simulink model "behavior_IMM_Pred"  (R2019b)
settings: Solver=FixedStepAuto  StartTime=0.0  StopTime=25  FixedStep=Ts_bp  RelTol=1e-3
undefined symbols (not defined in the file or in its folder): P_init, sigbuilder_block, Ts_bp, vx, vy, x, y
libraries: simulink x2
settings Model: Creator=jasprit  LastModifiedBy=jasprit

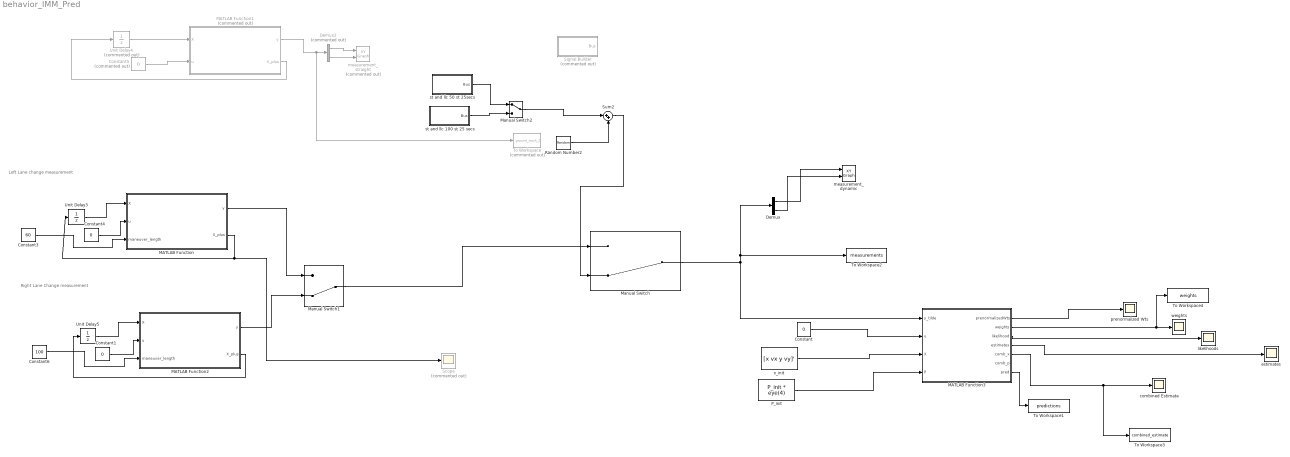
== system behavior_IMM_Pred ==
  note: Left Lane change measurement
  note: Right Lane Change measurement
  Constant : Constant  Value=0
  Constant1 : Constant  Value=0  SampleTime=-1
  Constant3 : Constant  Value=60  SampleTime=-1
  Constant4 : Constant  Value=0  SampleTime=-1
  Constant5 : Constant  Commented=on  Value=0  SampleTime=-1
  Constant6 : Constant  Value=100  SampleTime=-1
  Demux : Demux  Outputs=2
  Demux2 : Demux  Commented=on  Outputs=2
  MATLAB Function : MATLAB Function  TreatAsAtomicUnit=on
  MATLAB Function1 : MATLAB Function  Commented=on  TreatAsAtomicUnit=on
  MATLAB Function2 : MATLAB Function  TreatAsAtomicUnit=on
  MATLAB Function3 : MATLAB Function  TreatAsAtomicUnit=on
  Manual Switch : ManualSwitch  CurrentSetting=0
  Manual Switch1 : ManualSwitch  CurrentSetting=0
  Manual Switch2 : ManualSwitch
  P_init : Constant  Value=P_init * eye(4)  SampleTime=-1
  Random Number2 : RandomNumber  Variance=0.0025  SampleTime=Ts_bp
  Scope : Scope  Commented=on
  Signal Builder : Subsystem  Tag=STV Subsys  Commented=on  LoadFcn=sigbuilder_block('load');  StartFcn=sigbuilder_block('start');  StopFcn=sigbuilder_block('stop');  ClipboardFcn=sigbuilder_block('clipboard');  mask(Sigbuilder block){tuvar=[0:10]}
      mask help: Simulink:masks:SigbuilderBlock_MD
      mask init:
      | if ~strcmp(get_param(bdroot(gcbh),'SimulationStatus'),'stopped') tuvar = sigbuilder_block('maskInit'); end
      settings: CopyFcn=sigbuilder_block('copy');  DeleteFcn=sigbuilder_block('delete');  ModelCloseFcn=sigbuilder_block('modelClose');  PreSaveFcn=sigbuilder_block('preSave');  PauseFcn=sigbuilder_block('pause');  ContinueFcn=sigbuilder_block('continue');  NameChangeFcn=sigbuilder_block('namechange');  OpenFcn=sigbuilder_block('open',[411 7.5 573 467.25 ]);  CloseFcn=sigbuilder_block('close');
      mask Display: plot(0, 0, 100, 100,[2, 2, 32, 32, 2], [68, 8, 8, 68, 68],[32, 2], [38, 38], [32, 19, 2],[53, 60, 44], [32, 17, 17, 2],[16, 16, 31, 31]);txt = getActiveGroup(gcbh);text(2, 100, txt,'verticalAlignment', 'top');
  Sum2 : Sum  Inputs=|++
  To Workspace : ToWorkspace  Commented=on  VariableName=ground_truth_2  SaveFormat=Timeseries  SampleTime=-1
  To Workspace1 : ToWorkspace  VariableName=predictions  SaveFormat=Timeseries  SampleTime=-1
  To Workspace2 : ToWorkspace  VariableName=measurements  SaveFormat=Timeseries  SampleTime=-1
  To Workspace3 : ToWorkspace  VariableName=combined_estimate  SaveFormat=Timeseries  SampleTime=-1
  To Workspace4 : ToWorkspace  VariableName=weights  SaveFormat=Timeseries  SampleTime=-1
  Unit Delay3 : UnitDelay  InitialCondition=[x vx y vy]  SampleTime=Ts_bp  HasFrameUpgradeWarning=on
  Unit Delay4 : UnitDelay  Commented=on  InitialCondition=[x vx y vy]  SampleTime=-1  HasFrameUpgradeWarning=on
  Unit Delay5 : UnitDelay  InitialCondition=[x vx y vy]  SampleTime=Ts_bp  HasFrameUpgradeWarning=on
  combined Estimate : Scope
  estimates : Scope
  likelihoods : Scope
  measurement_dynamic : simulink/Sinks/XY Graph  xmin=-1  xmax=200  ymin=-5  ymax=5  st=-1
  measurement_straight : simulink/Sinks/XY Graph  Commented=on  xmin=-1  xmax=200  ymin=-5  ymax=5  st=-1
  prenormalized Wts : Scope
  st and llc 100 st 25 secs : Subsystem  Tag=STV Subsys  LoadFcn=sigbuilder_block('load');  StartFcn=sigbuilder_block('start');  StopFcn=sigbuilder_block('stop');  ClipboardFcn=sigbuilder_block('clipboard');  mask(Sigbuilder block){tuvar=[0:10]}
      mask help: Simulink:masks:SigbuilderBlock_MD
      mask init:
      | if ~strcmp(get_param(bdroot(gcbh),'SimulationStatus'),'stopped') tuvar = sigbuilder_block('maskInit'); end
      settings: CopyFcn=sigbuilder_block('copy');  DeleteFcn=sigbuilder_block('delete');  ModelCloseFcn=sigbuilder_block('modelClose');  PreSaveFcn=sigbuilder_block('preSave');  PauseFcn=sigbuilder_block('pause');  ContinueFcn=sigbuilder_block('continue');  NameChangeFcn=sigbuilder_block('namechange');  OpenFcn=sigbuilder_block('open',[437.25 157.5 550.5 399.75 ]);  CloseFcn=sigbuilder_block('close');
      mask Display: plot(0, 0, 100, 100,[2, 2, 32, 32, 2], [68, 8, 8, 68, 68],[32, 2], [38, 38], [32, 19, 2],[53, 60, 44], [32, 17, 17, 2],[16, 16, 31, 31]);txt = getActiveGroup(gcbh);text(2, 100, txt,'verticalAlignment', 'top');
  st and llc 50 st 25secs : Subsystem  Tag=STV Subsys  LoadFcn=sigbuilder_block('load');  StartFcn=sigbuilder_block('start');  StopFcn=sigbuilder_block('stop');  ClipboardFcn=sigbuilder_block('clipboard');  mask(Sigbuilder block){tuvar=[0:10]}
      mask help: Simulink:masks:SigbuilderBlock_MD
      mask init:
      | if ~strcmp(get_param(bdroot(gcbh),'SimulationStatus'),'stopped') tuvar = sigbuilder_block('maskInit'); end
      settings: CopyFcn=sigbuilder_block('copy');  DeleteFcn=sigbuilder_block('delete');  ModelCloseFcn=sigbuilder_block('modelClose');  PreSaveFcn=sigbuilder_block('preSave');  PauseFcn=sigbuilder_block('pause');  ContinueFcn=sigbuilder_block('continue');  NameChangeFcn=sigbuilder_block('namechange');  OpenFcn=sigbuilder_block('open',[433.5 132.75 558 422.25 ]);  CloseFcn=sigbuilder_block('close');
      mask Display: plot(0, 0, 100, 100,[2, 2, 32, 32, 2], [68, 8, 8, 68, 68],[32, 2], [38, 38], [32, 19, 2],[53, 60, 44], [32, 17, 17, 2],[16, 16, 31, 31]);txt = getActiveGroup(gcbh);text(2, 100, txt,'verticalAlignment', 'top');
  weights : Scope
  x_init : Constant  Value=[x vx y vy]'
  wires:
  Unit Delay3/1 -> MATLAB Function/1(X)
  MATLAB Function2/1(y) -> Manual Switch1/2
  Demux2/1 -> measurement_straight/1
  Constant/1 -> MATLAB Function3/2(u)
  Unit Delay5/1 -> MATLAB Function2/1(X)
  MATLAB Function1/1(y) -> To Workspace/1, Demux2/1
  Constant1/1 -> MATLAB Function2/2(u)
  Constant6/1 -> MATLAB Function2/3(maneuver_length)
  MATLAB Function/1(y) -> Manual Switch1/1
  Manual Switch/1 -> MATLAB Function3/1(y_tilde), Demux/1, To Workspace2/1
  Constant4/1 -> MATLAB Function/2(u)
  Unit Delay4/1 -> MATLAB Function1/1(X)
  Demux/1 -> measurement_dynamic/1
  Constant3/1 -> MATLAB Function/3(maneuver_length)
  MATLAB Function1/2(X_plus) -> Unit Delay4/1
  MATLAB Function/2(X_plus) -> Scope/1, Unit Delay3/1
  Sum2/1 -> Manual Switch/2
  Random Number2/1 -> Sum2/2
  Constant5/1 -> MATLAB Function1/2(u)
  MATLAB Function2/2(X_plus) -> Unit Delay5/1
  Demux2/2 -> measurement_straight/2
  Demux/2 -> measurement_dynamic/2
  Manual Switch1/1 -> Manual Switch/1
  P_init/1 -> MATLAB Function3/4(P)
  MATLAB Function3/1(prenormalizedWts) -> prenormalized Wts/1
  MATLAB Function3/2(weights) -> To Workspace4/1, weights/1
  MATLAB Function3/3(likelihood) -> likelihoods/1
  MATLAB Function3/4(estimates) -> estimates/1
  x_init/1 -> MATLAB Function3/3(X)
  MATLAB Function3/5(comb_x) -> To Workspace3/1, combined Estimate/1
  st and llc 100 st 25 secs/1(Bus) -> Manual Switch2/2
  Manual Switch2/1 -> Sum2/1
  st and llc 50 st 25secs/1(Bus) -> Manual Switch2/1
  MATLAB Function3/7(pred) -> To Workspace1/1

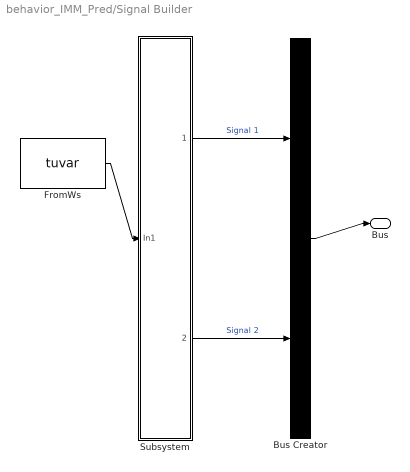
== system behavior_IMM_Pred/Signal Builder ==
  Bus Creator : BusCreator  Tag=Bus Creator  Inputs=2
  FromWs : FromWorkspace  Tag=STV FromWs  VariableName=tuvar  SampleTime=0
      SigBuilderData=|
      | common.afterFinalStr = 'Extrapolate'
      | common.sampleTime = 0
      | dataSet.timeRange = [0 20]
      | dataSet.name = 'Group 1'
      | sbobj.Groups.Name = 'Group 1'
      | sbobj.Groups.Signals(1).Name = 'Signal 1'
      | sbobj.Groups.Signals(1).XData = [0 0.01 0.02 0.03 0.04 0.05 0.06 0.07 0.08 0.09 0.1 0.11 ... (2001 elements, 1x2001)]
      | sbobj.Groups.Signals(1).YData = [0 0.1 0.2 0.3 0.4 0.5 0.6 0.7 0.8 0.9 1 1.1 ... (2001 elements, 1x2001)]
      | sbobj.Groups.Signals(2).Name = 'Signal 2'
      | sbobj.Groups.Signals(2).XData = [0 0.01 0.02 0.03 0.04 0.05 0.06 0.07 0.08 0.09 0.1 0.11 ... (2001 elements, 1x2001)]
      | sbobj.Groups.Signals(2).YData = [0 0 0 0 0 0 0 0 0 0 0 0 ... (2001 elements, 1x2001)]
      | sbobj.Groups.TimeRange = [0 20]
  Subsystem : Subsystem
  Bus : Outport  VectorParamsAs1DForOutWhenUnconnected=off
  wires:
  FromWs/1 -> Subsystem/1(In1)
  Bus Creator/1 -> Bus/1
  Subsystem/1(Signal 1) -> Bus Creator/1  "Signal 1"
  Subsystem/2(Signal 2) -> Bus Creator/2  "Signal 2"

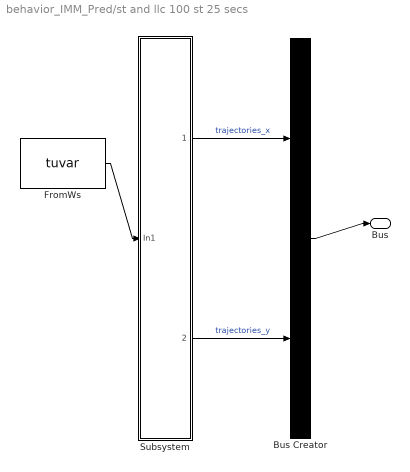
== system behavior_IMM_Pred/st and llc 100 st 25 secs ==
  Bus Creator : BusCreator  Tag=Bus Creator  Inputs=2
  FromWs : FromWorkspace  Tag=STV FromWs  VariableName=tuvar  SampleTime=0
      SigBuilderData=|
      | common.afterFinalStr = 'Extrapolate'
      | common.sampleTime = 0
      | dataSet.timeRange = [0 25]
      | dataSet.name = 'Group 1'
      | sbobj.Groups.Name = 'Group 1'
      | sbobj.Groups.Signals(1).Name = 'trajectories_x'
      | sbobj.Groups.Signals(1).XData = [0 0.01 0.02 0.03 0.04 0.05 0.06 0.07 0.08 0.09 0.1 0.11 ... (2501 elements, 1x2501)]
      | sbobj.Groups.Signals(1).YData = [0 0.1 0.2 0.3 0.4 0.5 0.6 0.7 0.8 0.9 1 1.1 ... (2501 elements, 1x2501)]
      | sbobj.Groups.Signals(2).Name = 'trajectories_y'
      | sbobj.Groups.Signals(2).XData = [0 0.01 0.02 0.03 0.04 0.05 0.06 0.07 0.08 0.09 0.1 0.11 ... (2501 elements, 1x2501)]
      | sbobj.Groups.Signals(2).YData = [0 0 0 0 0 0 0 0 0 0 0 0 ... (2501 elements, 1x2501)]
      | sbobj.Groups.TimeRange = [0 25]
  Subsystem : Subsystem
  Bus : Outport
  wires:
  FromWs/1 -> Subsystem/1(In1)
  Subsystem/1(trajectories_x) -> Bus Creator/1  "trajectories_x"
  Subsystem/2(trajectories_y) -> Bus Creator/2  "trajectories_y"
  Bus Creator/1 -> Bus/1

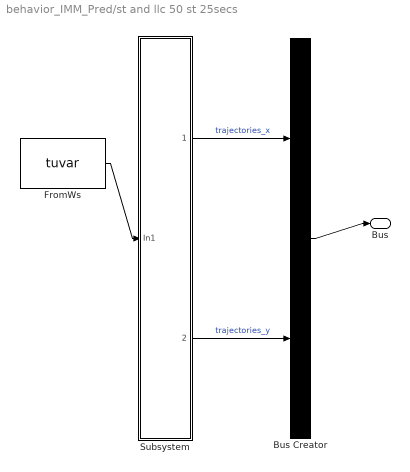
== system behavior_IMM_Pred/st and llc 50 st 25secs ==
  Bus Creator : BusCreator  Tag=Bus Creator  Inputs=2
  FromWs : FromWorkspace  Tag=STV FromWs  VariableName=tuvar  SampleTime=0
      SigBuilderData=|
      | common.afterFinalStr = 'Extrapolate'
      | common.sampleTime = 0
      | dataSet.timeRange = [0 25]
      | dataSet.name = 'Group 1'
      | sbobj.Groups.Name = 'Group 1'
      | sbobj.Groups.Signals(1).Name = 'trajectories_x'
      | sbobj.Groups.Signals(1).XData = [0 0.01 0.02 0.03 0.04 0.05 0.06 0.07 0.08 0.09 0.1 0.11 ... (2501 elements, 1x2501)]
      | sbobj.Groups.Signals(1).YData = [0 0.1 0.2 0.3 0.4 0.5 0.6 0.7 0.8 0.9 1 1.1 ... (2501 elements, 1x2501)]
      | sbobj.Groups.Signals(2).Name = 'trajectories_y'
      | sbobj.Groups.Signals(2).XData = [0 0.01 0.02 0.03 0.04 0.05 0.06 0.07 0.08 0.09 0.1 0.11 ... (2501 elements, 1x2501)]
      | sbobj.Groups.Signals(2).YData = [0 0 0 0 0 0 0 0 0 0 0 0 ... (2501 elements, 1x2501)]
      | sbobj.Groups.TimeRange = [0 25]
  Subsystem : Subsystem
  Bus : Outport
  wires:
  FromWs/1 -> Subsystem/1(In1)
  Subsystem/1(trajectories_x) -> Bus Creator/1  "trajectories_x"
  Subsystem/2(trajectories_y) -> Bus Creator/2  "trajectories_y"
  Bus Creator/1 -> Bus/1

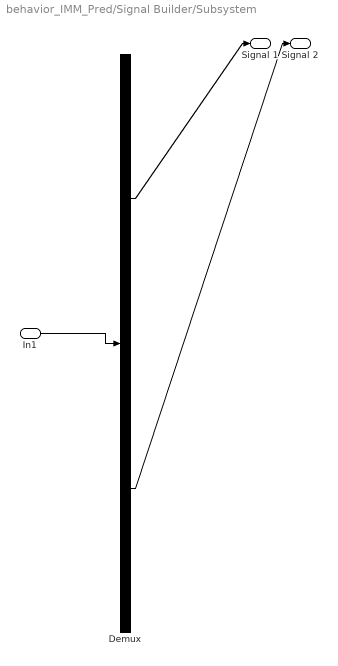
== system behavior_IMM_Pred/Signal Builder/Subsystem ==
  In1 : Inport
  Demux : Demux  Tag=STV Demux  Outputs=2
  Signal 1 : Outport  Tag=STV Outport  VectorParamsAs1DForOutWhenUnconnected=off
  Signal 2 : Outport  Tag=STV Outport  Port=2  VectorParamsAs1DForOutWhenUnconnected=off
  wires:
  In1/1 -> Demux/1
  Demux/1 -> Signal 1/1
  Demux/2 -> Signal 2/1

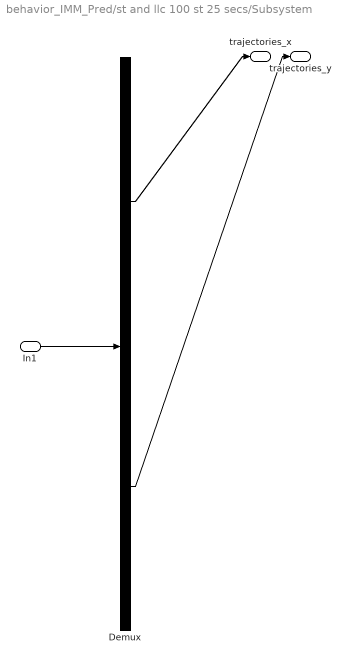
== system behavior_IMM_Pred/st and llc 100 st 25 secs/Subsystem ==
  In1 : Inport
  Demux : Demux  Tag=STV Demux  Outputs=2
  trajectories_x : Outport  Tag=STV Outport
  trajectories_y : Outport  Tag=STV Outport  Port=2
  wires:
  Demux/1 -> trajectories_x/1
  Demux/2 -> trajectories_y/1
  In1/1 -> Demux/1

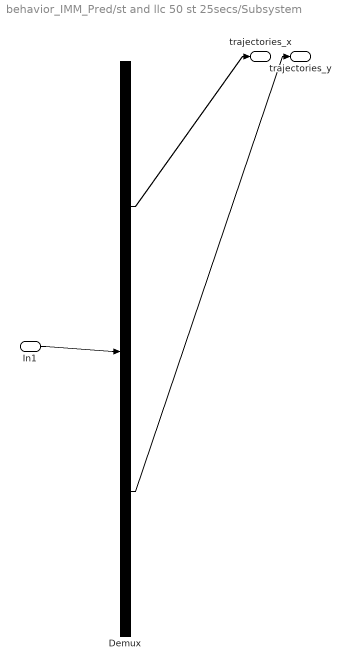
== system behavior_IMM_Pred/st and llc 50 st 25secs/Subsystem ==
  In1 : Inport
  Demux : Demux  Tag=STV Demux  Outputs=2
  trajectories_x : Outport  Tag=STV Outport
  trajectories_y : Outport  Tag=STV Outport  Port=2
  wires:
  Demux/1 -> trajectories_x/1
  Demux/2 -> trajectories_y/1
  In1/1 -> Demux/1

== matlab function behavior_IMM_Pred/MATLAB Function ==
  data: X input; u input; y output; X_plus output; maneuver_length input
function [y, X_plus]= measurementsForLaneChange(X, u, maneuver_length)

    Ts_bp = 0.1;
%     maneuver_length = 150;  %m
    lane_center_to_center_distance = 3.5;   %meters

    % states - X = [x vx y vy] -     
    Ck = [1 0 0 0; 0 0 1 0];

    % measurement noise std_dev
%     R_sigma = [0.5 0; 0 0.5];
   R_sigma = [0.05 0; 0 0.05];
    
    % process noise std dev
%    sigma_matrix = diag([0.16 0.16 0.16 0.16]);
    sigma_matrix = diag([0.032 0.032 0.032 0.032]);
    
%     if t < 15
%         Ak = [1 Ts 0 0; 0 1 0 0; 0 0 1 Ts; 0 0 0 1];
%         Bk = 0;
%         X_plus = Ak * X + Bk * u + sqrt(Ts) * sigma_matrix * randn(4,1);
%     else
        X_plus = leftLaneChangeParametricFcn(X, u, maneuver_length, lane_center_to_center_distance) + sqrt(Ts_bp)*sigma_matrix*randn(4,1);    
%     end
    
    y = Ck * X_plus + R_sigma * randn(2,1);
    
end

== matlab function behavior_IMM_Pred/MATLAB Function1 ==
  data: X input; u input; y output; X_plus output
function [y, X_plus]= measurementsForStraightMotion(X, u)

    Ts_bp = 0.1;
    % states - X = [x vx y vy] -     
    Ak = [1 Ts_bp 0 0; 0 1 0 0; 0 0 1 Ts_bp; 0 0 0 1];
    Bk = 0;
    Ck = [1 0 0 0; 0 0 1 0];

    % measurement noise std_dev
%     R_sigma = [0.5 0; 0 0.5];
   R_sigma = [0.05 0; 0 0.05];
    
    % process noise std dev
%    sigma_matrix = diag([0.16 0.16 0.16 0.16]);
    sigma_matrix = diag([0.032 0.032 0.032 0.032]);
  
    X(3) = 0;
%    X(4) = 0;
    
    X_plus = Ak * X + Bk * u + sqrt(Ts_bp)*sigma_matrix*randn(4,1);    
    
    y = Ck * X_plus + R_sigma * randn(2,1);
    
end

== matlab function behavior_IMM_Pred/MATLAB Function2 ==
  data: X input; u input; y output; X_plus output; maneuver_length input
function [y, X_plus]= measurementsForLaneChange(X, u, maneuver_length)

    Ts_bp = 0.1;
%    maneuver_length = 150;  %m
    lane_center_to_center_distance = 3.5;   %meters

    % states - X = [x vx y vy] -     
    Ck = [1 0 0 0; 0 0 1 0];

    % measurement noise std_dev
%     R_sigma = [0.5 0; 0 0.5];
   R_sigma = [0.05 0; 0 0.05];
    
    % process noise std dev
%    sigma_matrix = diag([0.16 0.16 0.16 0.16]);
    sigma_matrix = diag([0.032 0.032 0.032 0.032]);
    
%     if t < 15
%         Ak = [1 Ts 0 0; 0 1 0 0; 0 0 1 Ts; 0 0 0 1];
%         Bk = 0;
%         X_plus = Ak * X + Bk * u + sqrt(Ts) * sigma_matrix * randn(4,1);
%     else
        X_plus = rightLaneChangeParametricFcn(X, u, maneuver_length, lane_center_to_center_distance) + sqrt(Ts_bp)*sigma_matrix*randn(4,1);    
%     end
    
    y = Ck * X_plus + R_sigma * randn(2,1);
    
end

== matlab function behavior_IMM_Pred/MATLAB Function3 ==
  data: y_tilde input; u input; prenormalizedWts output; X input; P input; weights output; likelihood output; estimates output; comb_x output; comb_p output; pred output
function [prenormalizedWts, weights, likelihood, estimates, comb_x, comb_p, pred]   = imm_laneChanges(y_tilde, u, X, P)
    persistent amm;
    Ts = 0.1;
    if isempty(amm)
%         Ts = 0.1;
        
        amm = HighwayAllBehaviorsIMMPred(Ts);
    end
    prediction_time_horizon = 5;
    no_of_filters = 5;
    max_no_of_states = 5;
    pred = zeros(max_no_of_states, prediction_time_horizon/Ts, no_of_filters);

    % mix initial states for the current cycle first
    amm.mixEstimates();

    % predict
    amm.predict(u);
    
    % correct and update probabilistic weights
    amm.correct(y_tilde);
    
    % combined estimates
    [comb_x, comb_p] = amm.calculateCombinedEstimate();
    
    prenormalizedWts = amm.getFilterNonNormalizedWeights();
    weights = amm.getFilterWeights();
    likelihood = amm.getFilterLikelihoods();
    estimates = amm.getFilterEstimates();
    pred = amm.getPredictions();
end
